simulink model "dec"  (R2020a)
settings: Solver=VariableStepAuto  StartTime=0.0  StopTime=10.0  RelTol=1e-3
model workspace (MAT data in the model file):
  K = 25
settings Model: Creator=Sainquake  LastModifiedBy=Sainquake

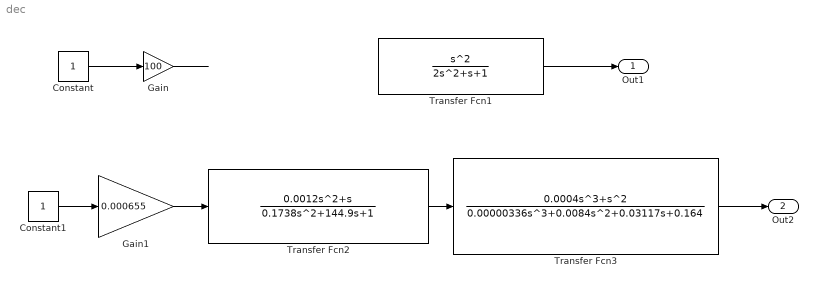
== system dec ==
  Constant : Constant
  Constant1 : Constant
  Gain : Gain  Gain=100
  Gain1 : Gain  Gain=0.000655
  Transfer Fcn1 : TransferFcn  Numerator=[1 0 0]  Denominator=[2 1 1]
  Transfer Fcn2 : TransferFcn  Numerator=[0.0012 1 0]  Denominator=[0.1738 144.9 1]
  Transfer Fcn3 : TransferFcn  Numerator=[0.0004 1 0 0]  Denominator=[0.00000336 0.0084 0.03117 0.164]
  Out1 : Outport
  Out2 : Outport  Port=2
  wires:
  Gain/1 -> ?
  ? -> Transfer Fcn1/1
  Transfer Fcn1/1 -> Out1/1
  Constant/1 -> Gain/1
  Transfer Fcn2/1 -> Transfer Fcn3/1
  Constant1/1 -> Gain1/1
  Gain1/1 -> Transfer Fcn2/1
  Transfer Fcn3/1 -> Out2/1
